simulink model "Lab2_22072026"  (R2019a)
settings: Solver=VariableStepAuto  StartTime=0.0  StopTime=0.5  RelTol=1e-3  EnableMultiTasking=on
settings Model: Creator=CSE  LastModifiedBy=Admin
settings DataIOCC: ReturnWorkspaceOutputs=off
settings OptimizationCC: LifeSpan=inf
settings DebuggingCC: SFUnexpectedBacktrackingDiag=warning  SFNoUnconditionalDefaultTransitionDiag=warning  ArithmeticOperatorsInVariantConditions=warning
settings SFSimCC: SimUseLocalCustomCode=off
settings RTWCC: RTWUseLocalCustomCode=off
settings CodeAppCC: StateflowObjectComments=on
settings GRTTargetCC: TargetLangStandard=C89/C90 (ANSI)  GeneratePreprocessorConditionals=Disable all
settings ConfigComp: CovMetricSettings=dw  CovHtmlReporting=on  CovSaveCumulativeToWorkspaceVar=on  CovSaveSingleToWorkspaceVar=on  CovExternalEMLEnable=off

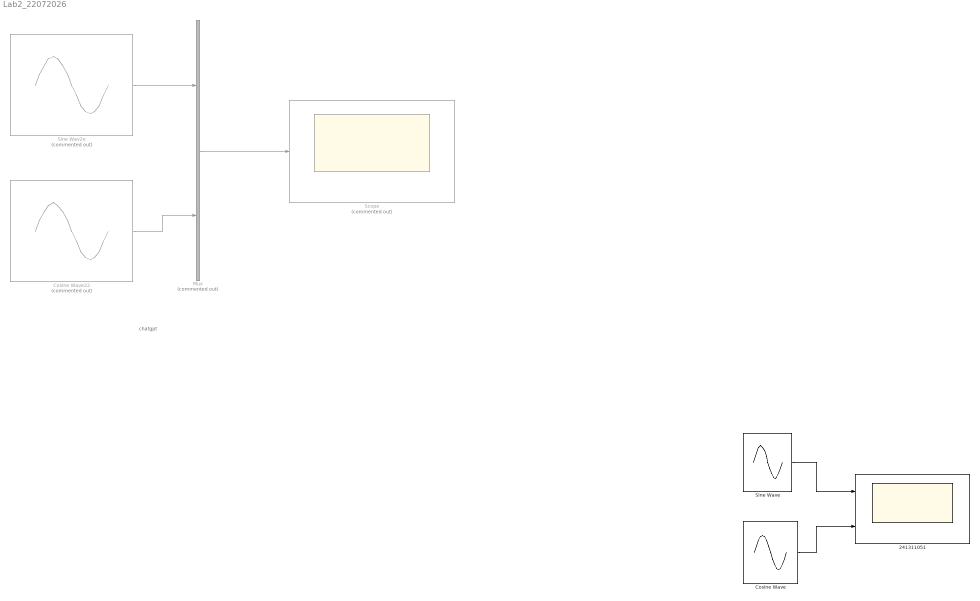
== system Lab2_22072026 ==
  note: chatgpt
  "241311051 " : Scope  NumInputPorts=2
  Cosine Wave : Sin  Frequency=2*pi*11  Phase=pi/2  SampleTime=1e-4
  Cosine Wave22 : Sin  Commented=on  Frequency=2*pi  Phase=pi/2  SampleTime=0
  Mux : Mux  Commented=on  Inputs=2
  Scope : Scope  Commented=on
  Sine Wav2e : Sin  Commented=on  Frequency=2*pi  SampleTime=0
  Sine Wave : Sin  Frequency=2*pi*21  SampleTime=1e-4
  wires:
  Sine Wav2e/1 -> Mux/1
  Cosine Wave22/1 -> Mux/2
  Mux/1 -> Scope/1
  Cosine Wave/1 -> "241311051 "/2
  Sine Wave/1 -> "241311051 "/1
